simulink model "GPG"  (R2019b)
settings: Solver=VariableStepAuto  StartTime=0.0  StopTime=20  RelTol=1e-3
libraries: dspmtrx3 x1, simulink x1
settings Model: Creator=gonz_jm  LastModifiedBy=gonz_jm
settings SolverCC: ZeroCrossAlgorithm=Adaptive
settings DebuggingCC: IgnoredZcDiagnostic=none

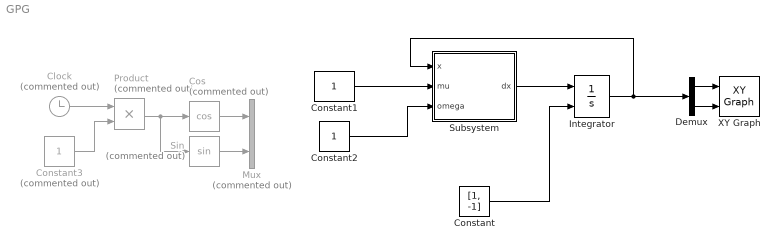
== system GPG ==
  Clock : Clock  Commented=on
  Constant : Constant  Value=[1, -1]
  Constant1 : Constant
  Constant2 : Constant
  Constant3 : Constant  Commented=on
  Cos : Trigonometry  Commented=on  Operator=cos
  Demux : Demux  Outputs=2
  Integrator : Integrator  InitialConditionSource=external
  Mux : Mux  Commented=on  Inputs=2
  Product : Product  Commented=on
  Sin : Trigonometry  Commented=on
  Subsystem : Subsystem
  XY Graph : simulink/Sinks/XY Graph  xmin=-2  xmax=2  ymin=-2  ymax=2  st=-1
  wires:
  Subsystem/1(dx) -> Integrator/1
  Constant/1 -> Integrator/2
  Integrator/1 -> Demux/1, Subsystem/1(x)
  Constant2/1 -> Subsystem/3(omega)
  Demux/1 -> XY Graph/1
  Demux/2 -> XY Graph/2
  Clock/1 -> Product/1
  Constant3/1 -> Product/2
  Product/1 -> Sin/1, Cos/1
  Cos/1 -> Mux/1
  Constant1/1 -> Subsystem/2(mu)
  Sin/1 -> Mux/2

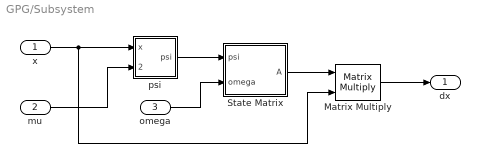
== system GPG/Subsystem ==
  x : Inport
  mu : Inport  Port=2
  omega : Inport  Port=3
  Matrix Multiply : Product  Multiplication=Matrix(*)
  State Matrix : Subsystem
  psi : Subsystem
  dx : Outport
  wires:
  State Matrix/1(A) -> Matrix Multiply/1
  x/1 -> psi/1(x), Matrix Multiply/2
  omega/1 -> State Matrix/2(omega)
  psi/1(psi) -> State Matrix/1(psi)
  mu/1 -> psi/2(mu)
  Matrix Multiply/1 -> dx/1

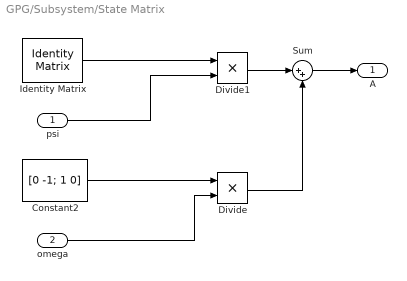
== system GPG/Subsystem/State Matrix ==
  psi : Inport
  omega : Inport  Port=2
  Constant2 : Constant  Value=[0 -1; 1 0]
  Divide : Product  Inputs=**
  Divide1 : Product  Inputs=**
  Identity Matrix : dspmtrx3/Identity Matrix  Inherit=off  N=2  Ts=1  dataType=double  isSigned=on  wordLen=16  udDataType=sfix(16)  fracBitsMode=Best precision  numFracBits=15  OutDataTypeStr=double  LastOutDataTypeStr=double
      settings: SourceProductName=DSP System Toolbox
  Sum : Sum  Inputs=|++
  A : Outport
  wires:
  psi/1 -> Divide1/2
  Constant2/1 -> Divide/1
  omega/1 -> Divide/2
  Divide1/1 -> Sum/1
  Divide/1 -> Sum/2
  Sum/1 -> A/1
  Identity Matrix/1 -> Divide1/1

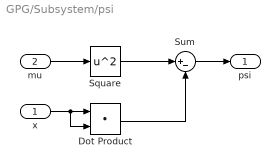
== system GPG/Subsystem/psi ==
  x : Inport
  mu : Inport  Port=2
  Dot Product : DotProduct  InputSameDT=on  OutDataTypeStr=Inherit: Inherit via internal rule
  Square : Math  Operator=square  SignedPower=off  SaturateOnIntegerOverflow=on
  Sum : Sum  Inputs=|+-
  psi : Outport
  wires:
  mu/1 -> Square/1
  Square/1 -> Sum/1
  x/1 -> Dot Product/2, Dot Product/1
  Dot Product/1 -> Sum/2
  Sum/1 -> psi/1
